simulink model "Simulacion_PID"  (R2017b)
settings: Solver=VariableStepAuto  StartTime=0.0  StopTime=350  RelTol=1e-3
settings Model: Creator=CPOH  LastModifiedBy=CPOH

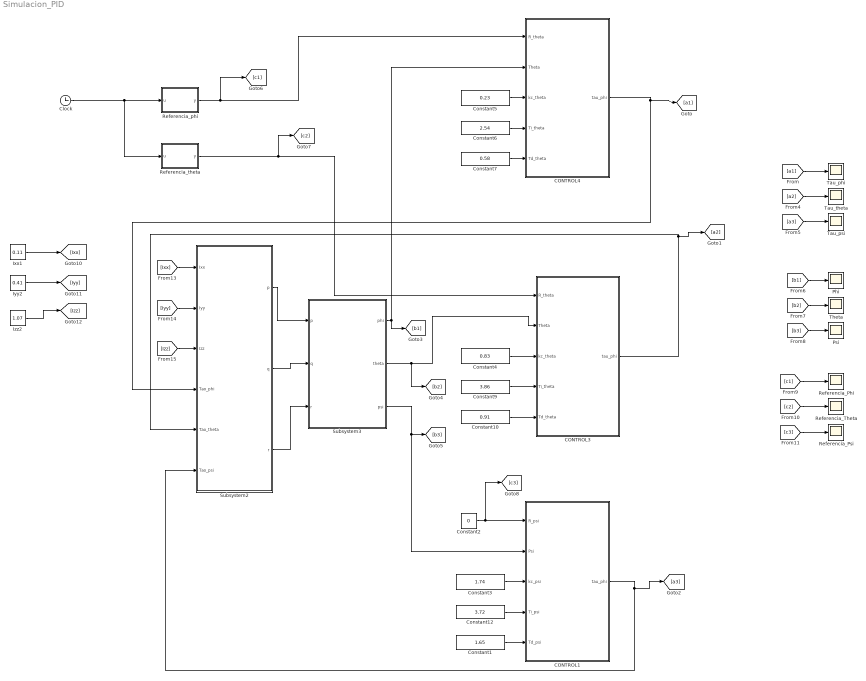
== system Simulacion_PID ==
  CONTROL1 : Subsystem
  CONTROL3 : Subsystem
  CONTROL4 : Subsystem
  Clock : Clock
  Constant1 : Constant  Value=1.65
  Constant10 : Constant  Value=0.91
  Constant12 : Constant  Value=3.72
  Constant2 : Constant  Value=0
  Constant3 : Constant  Value=1.74
  Constant4 : Constant  Value=0.83
  Constant5 : Constant  Value=0.23
  Constant6 : Constant  Value=2.54
  Constant7 : Constant  Value=0.58
  Constant9 : Constant  Value=3.86
  Ixx1 : Constant  Value=0.11
  Iyy2 : Constant  Value=0.41
  Izz2 : Constant  Value=1.07
  Phi : Scope
  Psi : Scope
  Referencia_Phi : Scope
  Referencia_Psi : Scope
  Referencia_Theta : Scope
  Referencia_phi : MATLAB Function  TreatAsAtomicUnit=on
  Referencia_theta : MATLAB Function  TreatAsAtomicUnit=on
  Subsystem2 : Subsystem
  Subsystem3 : Subsystem
  Tau_phi : Scope
  Tau_psi : Scope
  Tau_theta : Scope
  Theta : Scope
  wires:
  Constant12/1 -> CONTROL1/4(Ti_psi)
  [Izz] -> Subsystem2/3(Izz)
  Ixx1/1 -> [Ixx]
  Iyy2/1 -> [Iyy]
  CONTROL3/1(tau_phi) -> [a2], Subsystem2/5(Tao_theta)
  [Iyy] -> Subsystem2/2(Iyy)
  Subsystem2/1(p) -> Subsystem3/1(p)
  Referencia_theta/1(y) -> [c2], CONTROL3/1(R_theta)
  Constant3/1 -> CONTROL1/3(kc_psi)
  Subsystem3/3(psi) -> [b3], CONTROL1/2(Psi)
  Izz2/1 -> [Izz]
  Constant10/1 -> CONTROL3/5(Td_theta)
  Clock/1 -> Referencia_phi/1(u), Referencia_theta/1(u)
  CONTROL4/1(tau_phi) -> [a1], Subsystem2/4(Tao_phi)
  Subsystem3/2(theta) -> CONTROL3/2(Theta), [b2]
  Constant4/1 -> CONTROL3/3(kc_theta)
  Constant9/1 -> CONTROL3/4(Ti_theta)
  Referencia_phi/1(y) -> [c1], CONTROL4/1(R_theta)
  Constant6/1 -> CONTROL4/4(Ti_theta)
  Constant7/1 -> CONTROL4/5(Td_theta)
  Subsystem3/1(phi) -> CONTROL4/2(Theta), [b1]
  Subsystem2/2(q) -> Subsystem3/2(q)
  Constant1/1 -> CONTROL1/5(Td_psi)
  Constant5/1 -> CONTROL4/3(kc_theta)
  Subsystem2/3(r) -> Subsystem3/3(r)
  [Ixx] -> Subsystem2/1(Ixx)
  Constant2/1 -> [c3], CONTROL1/1(R_psi)
  [b1] -> Phi/1
  [c3] -> Referencia_Psi/1
  [c2] -> Referencia_Theta/1
  [b3] -> Psi/1
  [a2] -> Tau_theta/1
  [b2] -> Theta/1
  [a1] -> Tau_phi/1
  [c1] -> Referencia_Phi/1
  [a3] -> Tau_psi/1
  CONTROL1/1(tau_phi) -> [a3], Subsystem2/6("Tao_psi ")

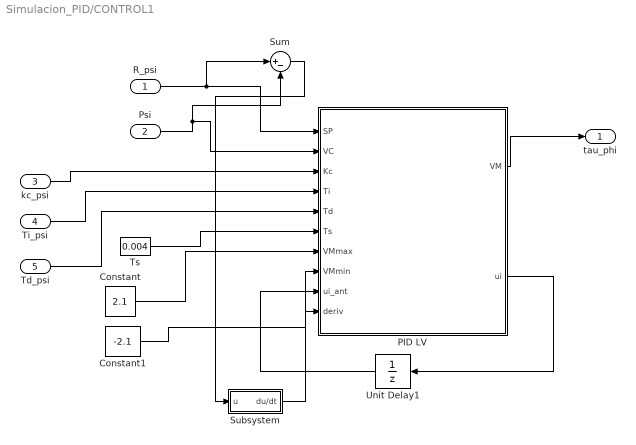
== system Simulacion_PID/CONTROL1 ==
  R_psi : Inport
  Psi : Inport  Port=2
  kc_psi : Inport  Port=3
  Ti_psi : Inport  Port=4
  Td_psi : Inport  Port=5
  Constant : Constant  Value=2.1
  Constant1 : Constant  Value=-2.1
  PID LV : MATLAB Function  TreatAsAtomicUnit=on
  Subsystem : Subsystem
  Sum : Sum  Inputs=|+-
  Ts : Constant  Value=0.004  SampleTime=0.004
  Unit Delay1 : UnitDelay  SampleTime=0.004
  tau_phi : Outport
  wires:
  Sum/1 -> Subsystem/1(u)
  Subsystem/1(du/dt) -> PID LV/10(deriv)
  Unit Delay1/1 -> PID LV/9(ui_ant)
  Constant1/1 -> PID LV/8(VMmin)
  PID LV/1(VM) -> tau_phi/1
  PID LV/2(ui) -> Unit Delay1/1
  Ts/1 -> PID LV/6(Ts)
  Psi/1 -> Sum/2, PID LV/2(VC)
  Constant/1 -> PID LV/7(VMmax)
  R_psi/1 -> Sum/1, PID LV/1(SP)
  kc_psi/1 -> PID LV/3(Kc)
  Ti_psi/1 -> PID LV/4(Ti)
  Td_psi/1 -> PID LV/5(Td)

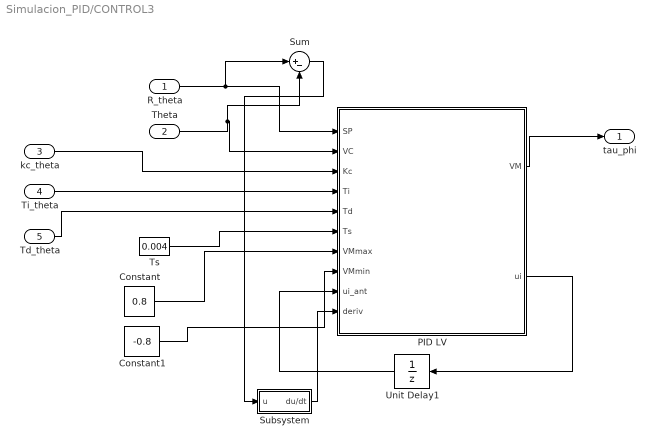
== system Simulacion_PID/CONTROL3 ==
  R_theta : Inport
  Theta : Inport  Port=2
  kc_theta : Inport  Port=3
  Ti_theta : Inport  Port=4
  Td_theta : Inport  Port=5
  Constant : Constant  Value=0.8
  Constant1 : Constant  Value=-0.8
  PID LV : MATLAB Function  TreatAsAtomicUnit=on
  Subsystem : Subsystem
  Sum : Sum  Inputs=|+-
  Ts : Constant  Value=0.004  SampleTime=0.004
  Unit Delay1 : UnitDelay  SampleTime=0.004
  tau_phi : Outport
  wires:
  Constant/1 -> PID LV/7(VMmax)
  Td_theta/1 -> PID LV/5(Td)
  R_theta/1 -> PID LV/1(SP), Sum/1
  Constant1/1 -> PID LV/8(VMmin)
  Theta/1 -> Sum/2, PID LV/2(VC)
  Ts/1 -> PID LV/6(Ts)
  Unit Delay1/1 -> PID LV/9(ui_ant)
  Sum/1 -> Subsystem/1(u)
  PID LV/1(VM) -> tau_phi/1
  Subsystem/1(du/dt) -> PID LV/10(deriv)
  PID LV/2(ui) -> Unit Delay1/1
  kc_theta/1 -> PID LV/3(Kc)
  Ti_theta/1 -> PID LV/4(Ti)

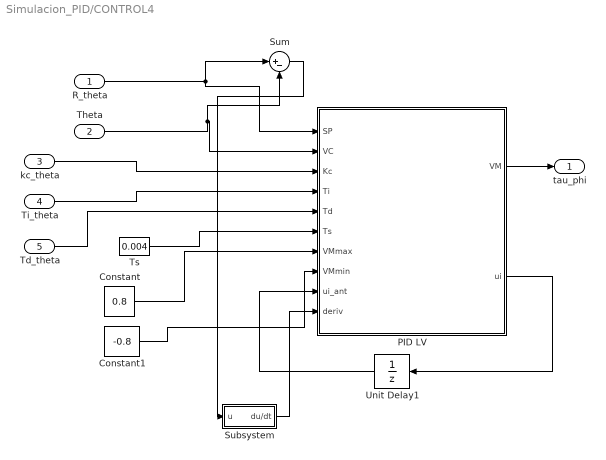
== system Simulacion_PID/CONTROL4 ==
  R_theta : Inport
  Theta : Inport  Port=2
  kc_theta : Inport  Port=3
  Ti_theta : Inport  Port=4
  Td_theta : Inport  Port=5
  Constant : Constant  Value=0.8
  Constant1 : Constant  Value=-0.8
  PID LV : MATLAB Function  TreatAsAtomicUnit=on
  Subsystem : Subsystem
  Sum : Sum  Inputs=|+-
  Ts : Constant  Value=0.004  SampleTime=0.004
  Unit Delay1 : UnitDelay  SampleTime=0.004
  tau_phi : Outport
  wires:
  Unit Delay1/1 -> PID LV/9(ui_ant)
  Theta/1 -> Sum/2, PID LV/2(VC)
  Constant/1 -> PID LV/7(VMmax)
  Sum/1 -> Subsystem/1(u)
  PID LV/1(VM) -> tau_phi/1
  PID LV/2(ui) -> Unit Delay1/1
  R_theta/1 -> PID LV/1(SP), Sum/1
  Subsystem/1(du/dt) -> PID LV/10(deriv)
  Constant1/1 -> PID LV/8(VMmin)
  Ts/1 -> PID LV/6(Ts)
  kc_theta/1 -> PID LV/3(Kc)
  Ti_theta/1 -> PID LV/4(Ti)
  Td_theta/1 -> PID LV/5(Td)

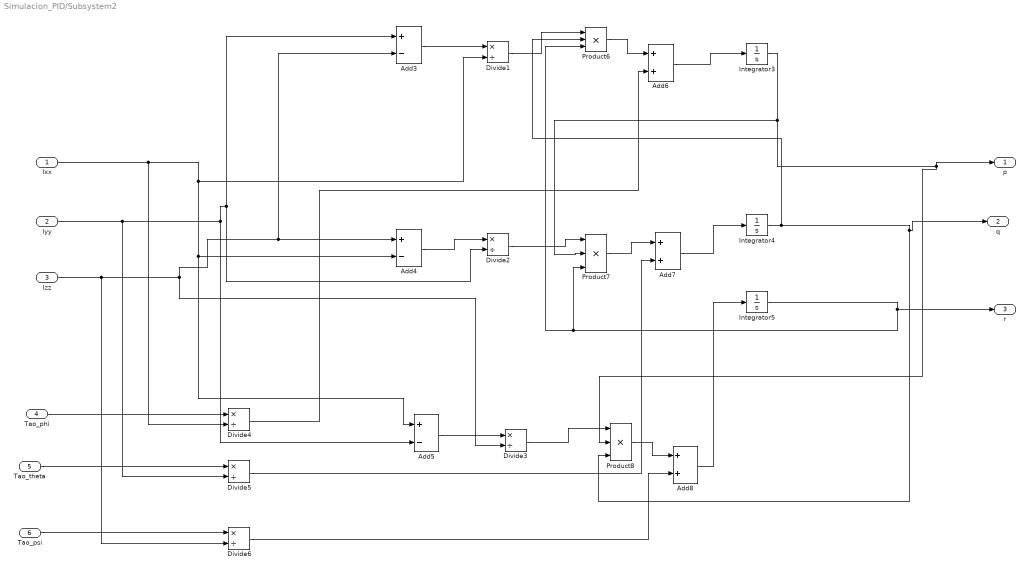
== system Simulacion_PID/Subsystem2 ==
  Ixx : Inport
  Iyy : Inport  Port=2
  Izz : Inport  Port=3
  Tao_phi : Inport  Port=4
  Tao_theta : Inport  Port=5
  "Tao_psi " : Inport  Port=6
  Add3 : Sum  Inputs=+-
  Add4 : Sum  Inputs=+-
  Add5 : Sum  Inputs=+-
  Add6 : Sum
  Add7 : Sum
  Add8 : Sum
  Divide{1..6} (6 alike) : Product  Inputs=*/
  Integrator3 : Integrator
  Integrator4 : Integrator
  Integrator5 : Integrator
  Product6 : Product  Inputs=3
  Product7 : Product  Inputs=3
  Product8 : Product  Inputs=3
  p : Outport
  q : Outport  Port=2
  r : Outport  Port=3
  wires:
  Divide3/1 -> Product8/1
  Divide2/1 -> Product7/1
  Product7/1 -> Add7/1
  Product6/1 -> Add6/1
  Add3/1 -> Divide1/1
  Add4/1 -> Divide2/1
  Divide1/1 -> Product6/1
  Tao_theta/1 -> Divide5/1
  Divide4/1 -> Add6/2
  Ixx/1 -> Divide1/2, Add4/2, Add5/1, Divide4/2
  Izz/1 -> Divide3/2, Add3/2, Add4/1, Divide6/2
  Tao_phi/1 -> Divide4/1
  Divide5/1 -> Add7/2
  "Tao_psi "/1 -> Divide6/1
  Divide6/1 -> Add8/2
  Integrator3/1 -> Product7/2, p/1, Product8/2
  Product8/1 -> Add8/1
  Integrator4/1 -> Product6/2, Product8/3, q/1
  Integrator5/1 -> Product6/3, Product7/3, r/1
  Add5/1 -> Divide3/1
  Add7/1 -> Integrator4/1
  Iyy/1 -> Add5/2, Divide2/2, Add3/1, Divide5/2
  Add6/1 -> Integrator3/1
  Add8/1 -> Integrator5/1

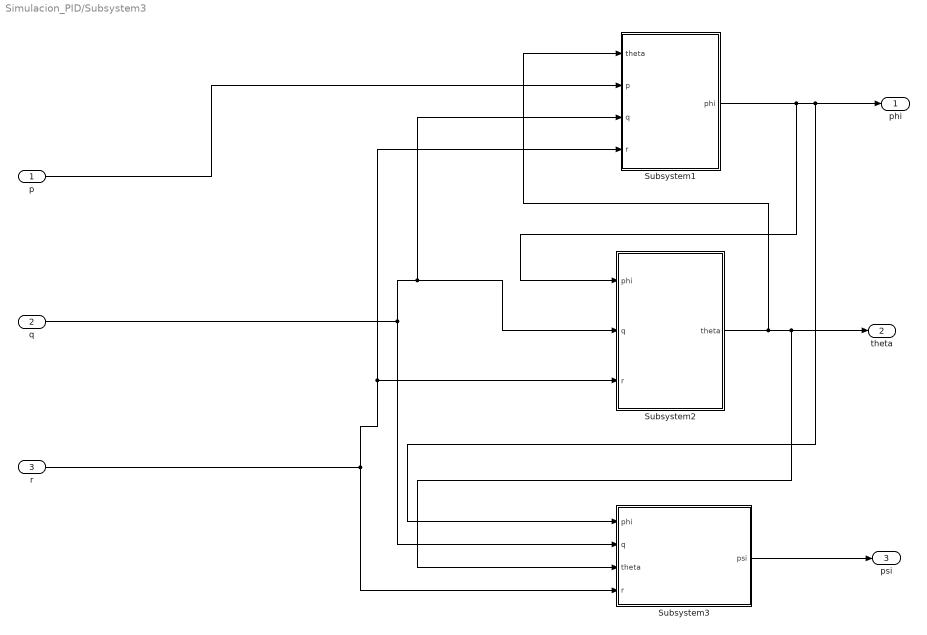
== system Simulacion_PID/Subsystem3 ==
  p : Inport
  q : Inport  Port=2
  r : Inport  Port=3
  Subsystem1 : Subsystem
  Subsystem2 : Subsystem
  Subsystem3 : Subsystem
  phi : Outport
  theta : Outport  Port=2
  psi : Outport  Port=3
  wires:
  Subsystem2/1(theta) -> Subsystem1/1(theta), Subsystem3/3(theta), theta/1
  Subsystem1/1(phi) -> Subsystem2/1(phi), Subsystem3/1(phi), phi/1
  p/1 -> Subsystem1/2(p)
  Subsystem3/1(psi) -> psi/1
  r/1 -> Subsystem3/4(r), Subsystem1/4(r), Subsystem2/3(r)
  q/1 -> Subsystem3/2(q), Subsystem1/3(q), Subsystem2/2(q)

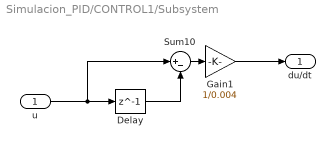
== system Simulacion_PID/CONTROL1/Subsystem ==
  u : Inport
  Delay : Delay  DelayLength=1  InitialCondition=0  SampleTime=0.004
  Gain1 : Gain  Gain=1/0.004  SampleTime=0.004
  Sum10 : Sum  Inputs=|+-
  du/dt : Outport
  wires:
  Gain1/1 -> du/dt/1
  Sum10/1 -> Gain1/1
  Delay/1 -> Sum10/2
  u/1 -> Delay/1, Sum10/1

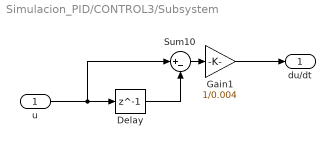
== system Simulacion_PID/CONTROL3/Subsystem ==
  u : Inport
  Delay : Delay  DelayLength=1  InitialCondition=0  SampleTime=0.004
  Gain1 : Gain  Gain=1/0.004  SampleTime=0.004
  Sum10 : Sum  Inputs=|+-
  du/dt : Outport
  wires:
  u/1 -> Sum10/1, Delay/1
  Delay/1 -> Sum10/2
  Sum10/1 -> Gain1/1
  Gain1/1 -> du/dt/1

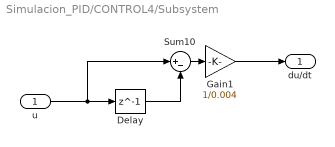
== system Simulacion_PID/CONTROL4/Subsystem ==
  u : Inport
  Delay : Delay  DelayLength=1  InitialCondition=0  SampleTime=0.004
  Gain1 : Gain  Gain=1/0.004  SampleTime=0.004
  Sum10 : Sum  Inputs=|+-
  du/dt : Outport
  wires:
  Gain1/1 -> du/dt/1
  Sum10/1 -> Gain1/1
  Delay/1 -> Sum10/2
  u/1 -> Delay/1, Sum10/1

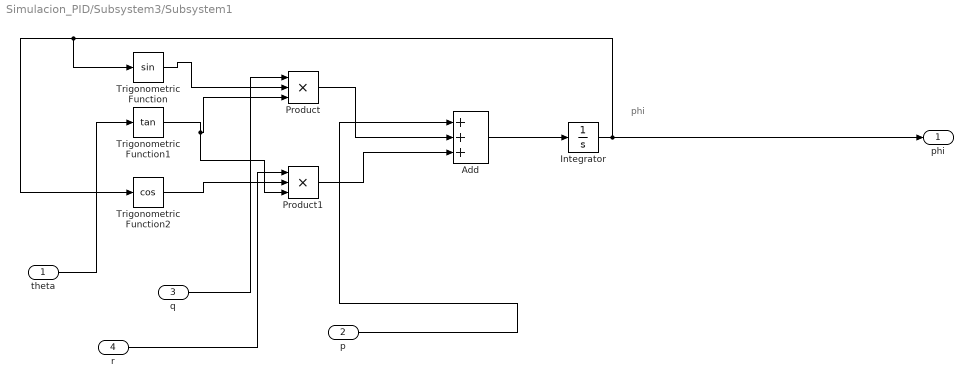
== system Simulacion_PID/Subsystem3/Subsystem1 ==
  note: phi
  theta : Inport
  p : Inport  Port=2
  q : Inport  Port=3
  r : Inport  Port=4
  Add : Sum  Inputs=+++
  Integrator : Integrator
  Product : Product  Inputs=3
  Product1 : Product  Inputs=3
  Trigonometric Function : Trigonometry
  Trigonometric Function1 : Trigonometry  Operator=tan
  Trigonometric Function2 : Trigonometry  Operator=cos
  phi : Outport
  wires:
  p/1 -> Add/1
  q/1 -> Product/1
  r/1 -> Product1/1
  Add/1 -> Integrator/1
  Trigonometric Function1/1 -> Product/3, Product1/3
  Trigonometric Function2/1 -> Product1/2
  Product/1 -> Add/2
  Trigonometric Function/1 -> Product/2
  Integrator/1 -> Trigonometric Function/1, Trigonometric Function2/1, phi/1
  Product1/1 -> Add/3
  theta/1 -> Trigonometric Function1/1

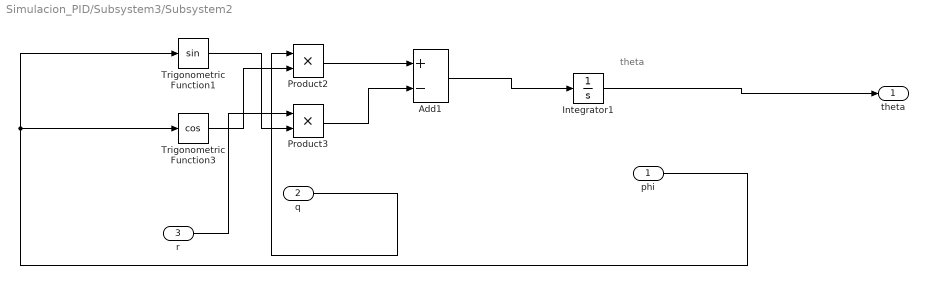
== system Simulacion_PID/Subsystem3/Subsystem2 ==
  note: theta
  phi : Inport
  q : Inport  Port=2
  r : Inport  Port=3
  Add1 : Sum  Inputs=+-
  Integrator1 : Integrator
  Product2 : Product
  Product3 : Product
  Trigonometric Function1 : Trigonometry
  Trigonometric Function3 : Trigonometry  Operator=cos
  theta : Outport
  wires:
  Trigonometric Function3/1 -> Product2/2
  Product2/1 -> Add1/1
  Add1/1 -> Integrator1/1
  Integrator1/1 -> theta/1
  Product3/1 -> Add1/2
  r/1 -> Product3/1
  phi/1 -> Trigonometric Function3/1, Trigonometric Function1/1
  q/1 -> Product2/1
  Trigonometric Function1/1 -> Product3/2

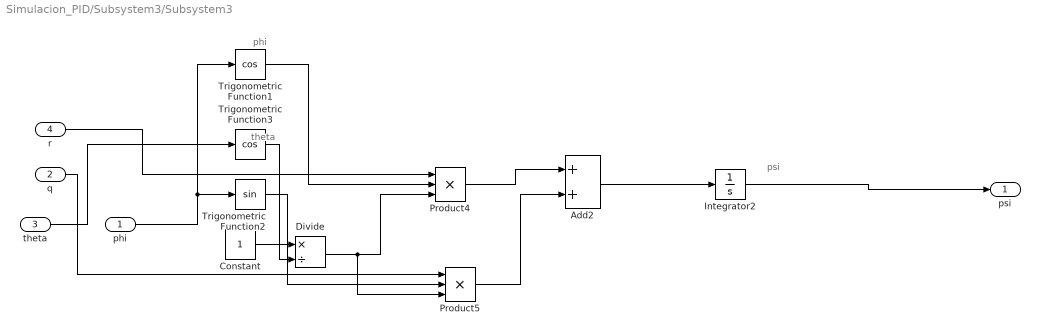
== system Simulacion_PID/Subsystem3/Subsystem3 ==
  note: psi
  note: phi
  note: theta
  phi : Inport
  q : Inport  Port=2
  theta : Inport  Port=3
  r : Inport  Port=4
  Add2 : Sum
  Constant : Constant
  Divide : Product  Inputs=*/
  Integrator2 : Integrator
  Product4 : Product  Inputs=3
  Product5 : Product  Inputs=3
  Trigonometric Function1 : Trigonometry  Operator=cos
  Trigonometric Function2 : Trigonometry
  Trigonometric Function3 : Trigonometry  Operator=cos
  psi : Outport
  wires:
  phi/1 -> Trigonometric Function1/1, Trigonometric Function2/1
  r/1 -> Product4/1
  theta/1 -> Trigonometric Function3/1
  q/1 -> Product5/1
  Constant/1 -> Divide/1
  Trigonometric Function2/1 -> Product5/2
  Product5/1 -> Add2/2
  Add2/1 -> Integrator2/1
  Trigonometric Function1/1 -> Product4/2
  Divide/1 -> Product4/3, Product5/3
  Product4/1 -> Add2/1
  Trigonometric Function3/1 -> Divide/2
  Integrator2/1 -> psi/1

== matlab function Simulacion_PID/CONTROL1/PID LV ==
  data: SP input; VM output; VC input; Kc input; Ti input; Td input; Ts input; VMmax input; VMmin input; ui_ant input; ui output; deriv input
function [VM,ui] = fcn(SP,VC,Kc,Ti,Td,Ts,VMmax,VMmin,ui_ant,deriv)


    
e=SP-VC;
%e_ant=ef_ant;

ui=0;
%ud=0;
u0=0;
feedforward=0;
N=0;

%Parte proporcional
up=Kc*e;

%Parte diferencial

ud=Kc*Td*deriv;


%Parte integral
if Ti==0
    ui=0;
else
ki=(Kc*Ts)/Ti;
 
ui=ui_ant+ki*e;
end

  VM=up+ui+ud+u0+feedforward;      
        

 %%%antiwindup
 if (VM<VMmin)
      VM=VMmin;
      ui=ui_ant;
 end
 if (VM>VMmax)
      VM=VMmax;
      ui=ui_ant;
 end

== matlab function Simulacion_PID/CONTROL3/PID LV ==
  data: SP input; VM output; VC input; Kc input; Ti input; Td input; Ts input; VMmax input; VMmin input; ui_ant input; ui output; deriv input
function [VM,ui] = fcn(SP,VC,Kc,Ti,Td,Ts,VMmax,VMmin,ui_ant,deriv)

   
e=SP-VC;
%e_ant=ef_ant;

ui=0;
%ud=0;
u0=0;
feedforward=0;
N=0;

%Parte proporcional
up=Kc*e;

%Parte diferencial

ud=Kc*Td*deriv;


%Parte integral
if Ti==0
    ui=0;
else
ki=(Kc*Ts)/Ti;
 
ui=ui_ant+ki*e;
end

  VM=up+ui+ud+u0+feedforward;      
        

 %%%antiwindup
 if (VM<VMmin)
      VM=VMmin;
      ui=ui_ant;
 end
 if (VM>VMmax)
      VM=VMmax;
      ui=ui_ant;
 end

== matlab function Simulacion_PID/CONTROL4/PID LV ==
  data: SP input; VM output; VC input; Kc input; Ti input; Td input; Ts input; VMmax input; VMmin input; ui_ant input; ui output; deriv input
function [VM,ui] = fcn(SP,VC,Kc,Ti,Td,Ts,VMmax,VMmin,ui_ant,deriv)



    
e=SP-VC;
%e_ant=ef_ant;

ui=0;
%ud=0;
u0=0;
feedforward=0;
N=0;

%Parte proporcional
up=Kc*e;

%Parte diferencial

ud=Kc*Td*deriv;


%Parte integral
if Ti==0
    ui=0;
else
ki=(Kc*Ts)/Ti;
 
ui=ui_ant+ki*e;
end

  VM=up+ui+ud+u0+feedforward;      
        

 %%%antiwindup
 if (VM<VMmin)
      VM=VMmin;
      ui=ui_ant;
 end
 if (VM>VMmax)
      VM=VMmax;
      ui=ui_ant;
 end

== matlab function Simulacion_PID/Referencia_phi ==
  data: u input; y output
function y = fcn(u)
offset2=120;
e=0;
if u>139.9-offset2
 e=0.2;   
end

if u>210.1-offset2
     e=-0.2;  
end

if u>272.2-offset2
     e=0;  
end

if u>327.2-offset2
    e=-0.3;
end

if u>366.3-offset2
    e=0.1;
end

if u>420.71-offset2
    e=0;
end




y = e;

== matlab function Simulacion_PID/Referencia_theta ==
  data: u input; y output
function y = fcn(u)
e=0;
offset2=120;
if u>139.9-offset2
 e=-0.3;   
end

if u>210.1-offset2
     e=0.1;  
end

if u>272.2-offset2
     e=0;  
end

if u>327.2-offset2
    e=0.2;
end

if u>366.3-offset2
    e=-0.2;
end

if u>420.71-offset2
    e=0;
end



y = e;
